simulink model "gbyk_rwd_tgtprob_countprob"  (R2015a)
settings: Solver=ode4  SolverMode=MultiTasking  StartTime=0.0  StopTime=inf  FixedStep=BKIN_STEP_TIME  RelTol=1e-3
StartFcn:
  |  warndlg('Dexterit-E models cannot run under simulation. Please compile your model and run it from within Dexterit-E.');set_param(bdroot,'SimulationCommand','stop')
model workspace (MAT data in the model file):
  BKIN_STEP_TIME = 0.00025
  col_x = 1
  col_y = 2
  INIT_COLOR = 5
  DELAY_POST_TRIAL = 8
  BKIN_KINEMATIC_FRAME_SIZE = 400
  HIT_COLOR = 6
  E_NO_EVENT = 0
  START_TARGET_COL = 1
  TARGET1_COL = 2
  TARGET2_COL = 3
  RWD_TARGET1_COL = 4
  RWD_TARGET2_COL = 5
  MAX_REACH_TIME_COL = 7
  K_DELAY_FIXED = 3
  K_DELAY_RAND = 4
  K_TRIGGER_VEL = 5
  K_TRIGGER_POS = 6
  K_THRESH_VELMAX = 7
  E_NEW_TRIAL = 1
  E_STAY_START = 2
  E_TARGET_TRIGGER = 5
  E_HIT_TARGET = 10
  E_MISS_TARGET = 11
  K_REWARD_VAL = 1
  VISUAL_RADIUS = 3
  LOGICAL_RADIUS = 4
  STROKE_WIDTH = 7
  TEXT_COLOR = 8
  LABEL_HEIGHT = 10
  E_TOO_SLOW = 20
  K_SCORETEXT_ROW = 2
  LABEL = 9
  E_TARGETS_ON = 3
  DISPLAY_TRIAL_COL = 9
  E_SHOW_INSTRUCT = 25
  E_SHOW_SCORE = 26
  INSTRUCT_PAUSE_BTN = 2
  TARGET1_PROB_COL = 6
  LABELONLY_X = 11
  LABELONLY_Y = 12
  K_PRE_REWARD_DELAY = 11
  K_RWDRATIO_5_8THS = 8
  K_RWDRATIO_6_8THS = 9
  K_RWDRATIO_7_8THS = 10
undefined symbols (not defined in the file or in its folder): slselsubs
libraries: slrtlib x8, Video x6, General x3, KINARM_general x3, simulink x2, xpcnilib x1
(part 2 of 2)

== matlab function gbyk_rwd_tgtprob_countprob/DisplayText/MATLAB Function ==
  data: VCODE input; score_dbl input; VCODE_mod output; fdbk_text input
function VCODE_mod = fcn(VCODE,score_dbl,fdbk_text)


VCODE_mod = VCODE;

score = round(score_dbl);  %for display purposes, round fractional rewards

if (fdbk_text == 0)  %if this is zero, show the score
       
    
    %score is in cents. potentially need to convert to dollars
    
    if (score < 10)
        text1 = 'You earned ';
        text2 = ' cents!';
        
        textout = [text1 int2char(int32(score)) text2];
        
    elseif (score < 100) %score < $1
        text1 = 'You earned ';
        text2 = ' cents!';
        
        n1 = int32(floor(double(score)/10));  %we need to cast score to a double otherwise the arithmetic is wrong!
        n2 = score - n1*10;
        
        textout = [text1 int2char(int32(n1)) int2char(int32(n2)) text2];
        
    else %score > $1, convert to dollars to keep the score readable
        text1 = 'You earned $';
        text2 = '.';
        text3 = '!';
        
        dollars = int32(floor(double(score)/100));
        if (dollars >= 10) %double digit dollar value
            n1d = int32(floor(double(dollars)/10));
            n2d = dollars - n1d*10;
            textdollars = [int2char(int32(n1d)) int2char(int32(n2d))];
        else %single digit
            textdollars = int2char(int32(dollars));
        end
        
        cents = score-dollars*100;
        if (cents < 10)
            textcents = ['0' int2char(int32(cents))];
        else
            n1 = int32(floor(double(cents)/10));
            n2 = round(cents - n1*10);
            textcents = [int2char(int32(n1)) int2char(int32(n2))];
        end
        
        textout = [text1 textdollars text2 textcents text3];
        
    end
    
elseif (fdbk_text == 1) 
    %print "too fast"
    textout = 'Too Fast!';
    
    
elseif (fdbk_text == 2) 
    %print "too fast"
    textout = 'Too Early!';

elseif (fdbk_text == -1) 
    %print "too slow"
    
    textout = 'Too Slow!';

elseif (fdbk_text == -2) 
    %print "too fast"
    textout = 'Too Late!';


else
    textout = '';
    
end
    

%the first character is VCODE(15)
%need to translate text into ascii:
textnum = double(textout); %this quickly casts each char into a number

%make sure we won't overflow the VCODE: no more than 50 chars! we will
%clip off anything that overflows.
VCODE_mod(1,15:min([15+length(textout),64])) = textnum(1:min([length(textnum),50])); %write out as many the characters as possible into the VCODE
VCODE_mod(1,min([15+length(textout)+1,64])) = 0;  %terminate the string!



function s = int2char(n)

n = mod(n,10); %make sure we only have 1 digit or we will get a weird character!

s = char(n+int32('0')); %// add the character
